simulink model "GES_Predictor"  (R2024a)
settings: Solver=VariableStepAuto  StartTime=0.0  StopTime=60  RelTol=1e-3
undefined symbols (not defined in the file): C_D, C_L, displacement, eta, magnitude, sail_area, turbine_area, wetted_area, wind_speed, zeta
settings Model: PacingRate=1.100000  Creator=energyship2  LastModifiedBy=energyship2

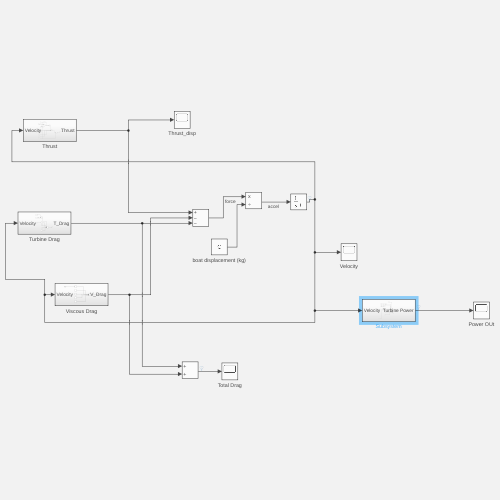
[thumbnail: Simulink's stored preview of the top-level diagram]
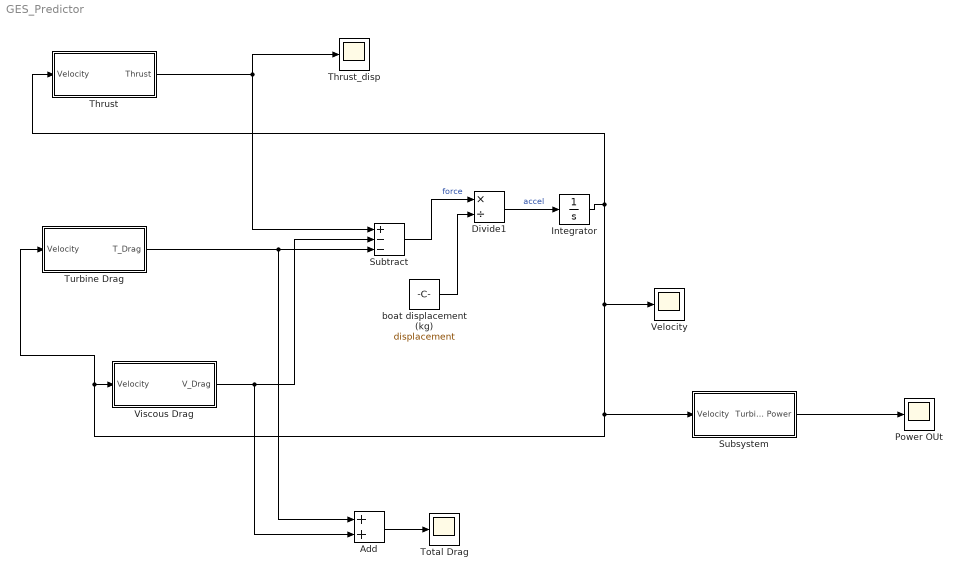
== system GES_Predictor ==
  Add : Sum
  Divide1 : Product  Inputs=*/
  Integrator : Integrator  LimitOutput=on
  Power OUt : Scope
  Subsystem : Subsystem
  Subtract : Sum  Inputs=+--
  Thrust : Subsystem
  Thrust_disp : Scope
  Total Drag : Scope
  Turbine Drag : Subsystem
  Velocity : Scope
  Viscous Drag : Subsystem
  boat displacement (kg) : Constant  Value=displacement
  wires:
  boat displacement (kg)/1 -> Divide1/2
  Subtract/1 -> Divide1/1  "force"
  Thrust/1(Thrust) -> Subtract/1, Thrust_disp/1
  Viscous Drag/1(V_Drag) -> Add/2, Subtract/2
  Divide1/1 -> Integrator/1  "accel"
  Integrator/1 -> Velocity/1, Turbine Drag/1(Velocity), Viscous Drag/1(Velocity), Subsystem/1(Velocity), Thrust/1(Velocity)
  Turbine Drag/1(T_Drag) -> Add/1, Subtract/3
  Add/1 -> Total Drag/1
  Subsystem/1(Turbine Power) -> Power OUt/1

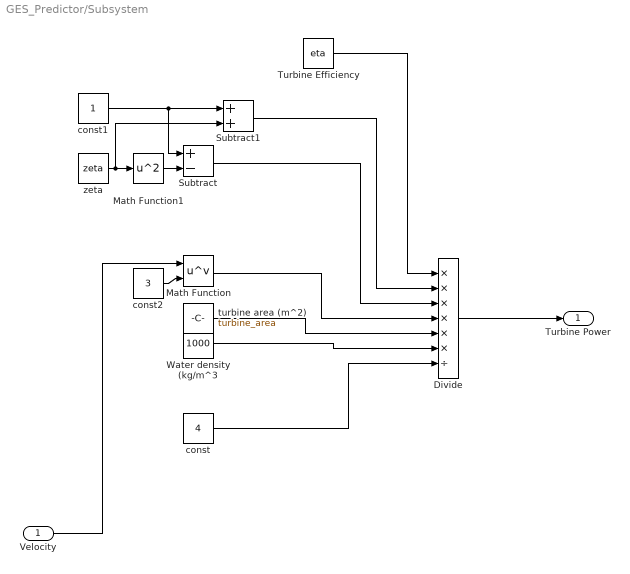
== system GES_Predictor/Subsystem ==
  Velocity : Inport
  Divide : Product  Inputs=******/
  Math Function : Math  Operator=pow
  Math Function1 : Math  Operator=square
  Subtract : Sum  Inputs=+-
  Subtract1 : Sum
  Turbine Efficiency : Constant  Value=eta
  Water density (kg/m^3 : Constant  Value=1000
  const : Constant  Value=4
  const1 : Constant
  const2 : Constant  Value=3
  turbine area (m^2) : Constant  Value=turbine_area
  zeta : Constant  Value=zeta
  Turbine Power : Outport
  wires:
  Math Function1/1 -> Subtract/2
  turbine area (m^2)/1 -> Divide/5
  Math Function/1 -> Divide/4
  const/1 -> Divide/7
  const1/1 -> Subtract1/1, Subtract/1
  Subtract/1 -> Divide/3
  zeta/1 -> Subtract1/2, Math Function1/1
  Velocity/1 -> Math Function/1
  Divide/1 -> Turbine Power/1
  Water density (kg/m^3/1 -> Divide/6
  const2/1 -> Math Function/2
  Subtract1/1 -> Divide/2
  Turbine Efficiency/1 -> Divide/1

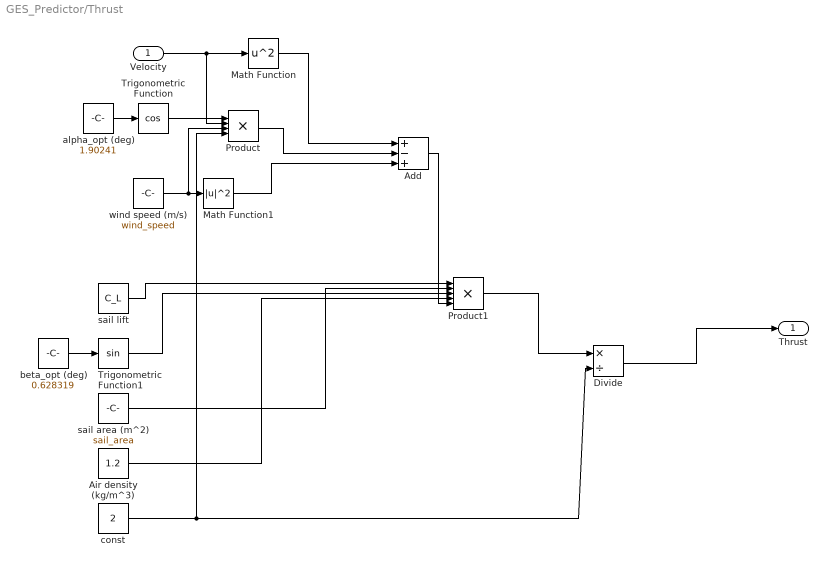
== system GES_Predictor/Thrust ==
  Velocity : Inport
  Add : Sum  Inputs=+-+
  Air density (kg/m^3) : Constant  Value=1.2
  Divide : Product  Inputs=*/
  Math Function : Math  Operator=square
  Math Function1 : Math  Operator=magnitude^2
  Product : Product  Inputs=4
  Product1 : Product  Inputs=5
  Trigonometric Function : Trigonometry  Operator=cos
  Trigonometric Function1 : Trigonometry
  alpha_opt (deg) : Constant  Value=1.90241
  beta_opt (deg) : Constant  Value=0.628319
  const : Constant  Value=2
  sail area (m^2) : Constant  Value=sail_area
  sail lift : Constant  Value=C_L
  wind speed (m/s) : Constant  Value=wind_speed
  Thrust : Outport
  wires:
  Velocity/1 -> Product/2, Math Function/1
  alpha_opt (deg)/1 -> Trigonometric Function/1
  beta_opt (deg)/1 -> Trigonometric Function1/1
  Math Function/1 -> Add/1
  wind speed (m/s)/1 -> Product/3, Math Function1/1
  Math Function1/1 -> Add/3
  Add/1 -> Product1/5
  Trigonometric Function/1 -> Product/1
  const/1 -> Divide/2, Product/4
  Product/1 -> Add/2
  sail area (m^2)/1 -> Product1/2
  Air density (kg/m^3)/1 -> Product1/4
  Trigonometric Function1/1 -> Product1/3
  sail lift/1 -> Product1/1
  Product1/1 -> Divide/1
  Divide/1 -> Thrust/1

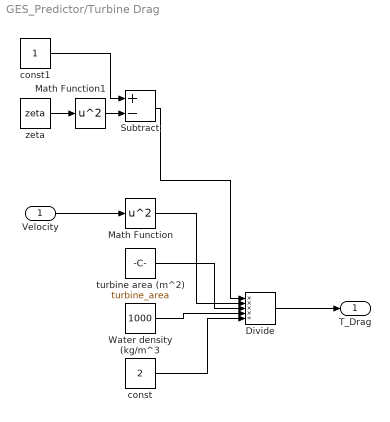
== system GES_Predictor/Turbine Drag ==
  Velocity : Inport
  Divide : Product  Inputs=****/
  Math Function : Math  Operator=square
  Math Function1 : Math  Operator=square
  Subtract : Sum  Inputs=+-
  Water density (kg/m^3 : Constant  Value=1000
  const : Constant  Value=2
  const1 : Constant
  turbine area (m^2) : Constant  Value=turbine_area
  zeta : Constant  Value=zeta
  T_Drag : Outport
  wires:
  Velocity/1 -> Math Function/1
  Water density (kg/m^3/1 -> Divide/4
  const/1 -> Divide/5
  turbine area (m^2)/1 -> Divide/3
  Math Function/1 -> Divide/2
  zeta/1 -> Math Function1/1
  Divide/1 -> T_Drag/1
  Math Function1/1 -> Subtract/2
  const1/1 -> Subtract/1
  Subtract/1 -> Divide/1

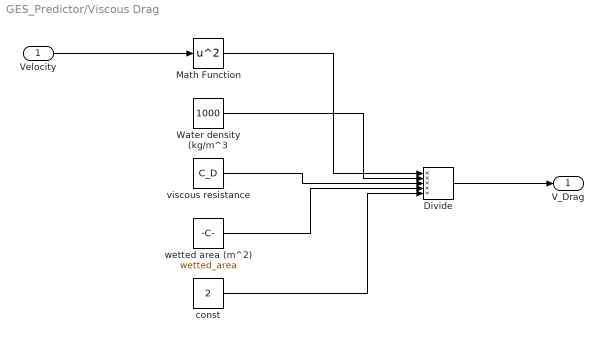
== system GES_Predictor/Viscous Drag ==
  Velocity : Inport
  Divide : Product  Inputs=****/
  Math Function : Math  Operator=square
  Water density (kg/m^3 : Constant  Value=1000
  const : Constant  Value=2
  viscous resistance : Constant  Value=C_D
  wetted area (m^2) : Constant  Value=wetted_area
  V_Drag : Outport
  wires:
  Velocity/1 -> Math Function/1
  Water density (kg/m^3/1 -> Divide/2
  const/1 -> Divide/5
  wetted area (m^2)/1 -> Divide/4
  Divide/1 -> V_Drag/1
  viscous resistance/1 -> Divide/3
  Math Function/1 -> Divide/1
